simulink model "CartPole_sim"  (R2018b)
settings: Solver=VariableStepAuto  StartTime=0.0  StopTime=100  FixedStep=0.005  MaxStep=0.005  RelTol=1e-3
libraries: neural x90
(part 3 of 3)

== system CartPole_sim/Controller/Layer 3/Delays 1 ==
  "p{3}" : Inport  PortDimensions=48
      mask Display: e = 0.06;c1 = [120 230 180]/255;c2 = ([120 230 180]+0)/(256+128);c3 = ([120 230 180]+128)/(256+128);patch([0 1 1 0],[0 0 1 1],c1);patch([0 1 1 1-e 1-e 0+e],[0 0 1 1-e 0+e 0+e],c2);patch([0 0 1 1-e 0+e 0+e],[0 1 1 1-e 1-e 0+e],c3);plot([0 1 1 0 0],[0 0 1 1 0]);
  mux : Mux  Inputs=1
      mask Display: e = 0.06;c1 = [120 150 230]/255;c2 = ([120 150 230]+0)/383;c3 = ([120 150 230]+128)/383;patch([0 1 1 0],[0 0 1 1],c1);patch([0 1 1 1-e 1-e 0+e],[0 0 1 1-e 0+e 0+e],c2);patch([0 0 1 1-e 0+e 0+e],[0 1 1 1-e 1-e 0+e],c3);plot([0 1 1 0 0],[0 0 1 1 0]);disp('Mux')
  "pd{3,2}" : Outport
      mask Display: e = 0.06;c1 = [120 230 180]/255;c2 = ([120 230 180]+0)/(256+128);c3 = ([120 230 180]+128)/(256+128);patch([0 1 1 0],[0 0 1 1],c1);patch([0 1 1 1-e 1-e 0+e],[0 0 1 1-e 0+e 0+e],c2);patch([0 0 1 1-e 0+e 0+e],[0 1 1 1-e 1-e 0+e],c3);plot([0 1 1 0 0],[0 0 1 1 0]);
  wires:
  mux/1 -> "pd{3,2}"/1
  "p{3}"/1 -> mux/1

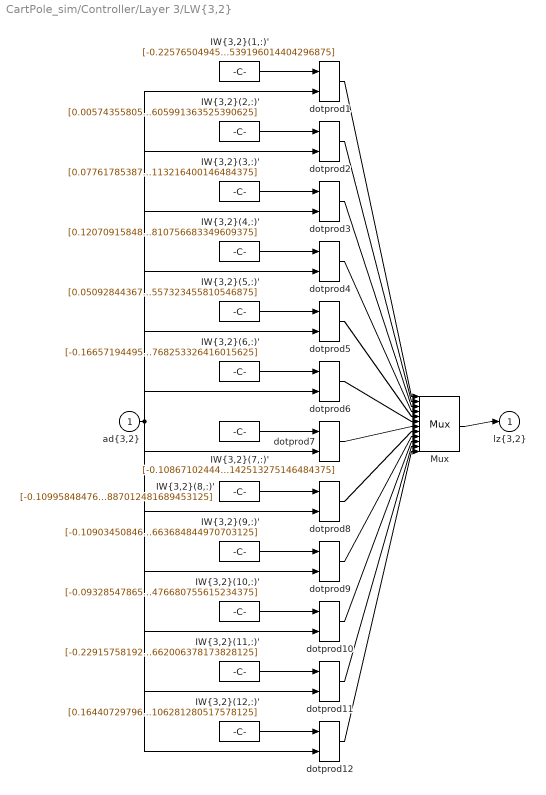
== system CartPole_sim/Controller/Layer 3/LW{3,2} ==
  "ad{3,2}" : Inport  PortDimensions=48
      mask Display: e = 0.06;c1 = [120 230 180]/255;c2 = ([120 230 180]+0)/(256+128);c3 = ([120 230 180]+128)/(256+128);patch([0 1 1 0],[0 0 1 1],c1);patch([0 1 1 1-e 1-e 0+e],[0 0 1 1-e 0+e 0+e],c2);patch([0 0 1 1-e 0+e 0+e],[0 1 1 1-e 1-e 0+e],c3);plot([0 1 1 0 0],[0 0 1 1 0]);
  "IW{3,2}(1,:)'" : Constant  Value=[-0.225765049457550048828125;0.70130741596221923828125;0.73611104488372802734375;0.85522115230560302734375;0.3625166416168212890625;-0.293086946010589599609375;-0.168597280979156494140625;0.62720489501953125;0.7177906036376953125;0.4205109775066375732421875;-0.22078745067119598388671875;0.786495685577392578125;0.598729610443115234375;0.857798099517822265625;-0.19783659279346466064453125;0.5886719226837158203125;0.033965639770030975341796875;0.4852178096771240234375;-0.4360056817531585693359375;-0.13498456776142120361328125;-0.2697825729846954345703125;0.6689045429229736328125;0.02779674716293811798095703125;0.2675172388553619384765625;0.789131581783294677734375;0.59786427021026611328125;0.614151060581207275390625;0.66306316852569580078125;0.59276866912841796875;-0.0609457008540630340576171875;0.62623417377471923828125;-0.18955354392528533935546875;0.755768299102783203125;-0.18641991913318634033203125;0.720268726348876953125;-0.0284832417964935302734375;1.03963196277618408203125;-0.119852729141712188720703125;0.10294115543365478515625;0.4573823511600494384765625;0.23938636481761932373046875;-0.16751043498516082763671875;0.67672908306121826171875;-0.668893158435821533203125;0.2460586130619049072265625;0.44056618213653564453125;0.53306019306182861328125;0.805462539196014404296875]
      mask Display: e = 0.06;c1 = [120 150 230]/255;c2 = ([120 150 230]+0)/383;c3 = ([120 150 230]+128)/383;patch([0 1 1 0],[0 0 1 1],c1);patch([0 1 1 1-e 1-e 0+e],[0 0 1 1-e 0+e 0+e],c2);patch([0 0 1 1-e 0+e 0+e],[0 1 1 1-e 1-e 0+e],c3);plot([0 1 1 0 0],[0 0 1 1 0]);disp('weights');
  "IW{3,2}(10,:)'" : Constant  Value=[-0.093285478651523590087890625;0.3607280552387237548828125;0.58088779449462890625;0.9831249713897705078125;0.71564197540283203125;0.21493326127529144287109375;-0.124086134135723114013671875;0.4439070522785186767578125;0.58334505558013916015625;0.3817100822925567626953125;-0.063464589416980743408203125;-0.2573592662811279296875;0.2025319039821624755859375;0.3065927028656005859375;0.32229793071746826171875;0.4737115204334259033203125;0.02929084934294223785400390625;0.1419357955455780029296875;-0.0101378001272678375244140625;0.3530226647853851318359375;0.707432687282562255859375;0.605476796627044677734375;-0.13292454183101654052734375;-0.0582952834665775299072265625;0.124955832958221435546875;0.519218027591705322265625;0.521830976009368896484375;0.083058618009090423583984375;0.1663186848163604736328125;0.2935204207897186279296875;0.5812957286834716796875;0.22234977781772613525390625;0.7579386234283447265625;0.0754846632480621337890625;0.3434390723705291748046875;-0.1704781055450439453125;0.21832014620304107666015625;-0.30861675739288330078125;-0.279193937778472900390625;0.10558624565601348876953125;0.85374772548675537109375;0.748513400554656982421875;0.553266108036041259765625;-0.24436579644680023193359375;0.08447755873203277587890625;0.507693231105804443359375;0.19571836292743682861328125;0.650114476680755615234375]
      mask Display: e = 0.06;c1 = [120 150 230]/255;c2 = ([120 150 230]+0)/383;c3 = ([120 150 230]+128)/383;patch([0 1 1 0],[0 0 1 1],c1);patch([0 1 1 1-e 1-e 0+e],[0 0 1 1-e 0+e 0+e],c2);patch([0 0 1 1-e 0+e 0+e],[0 1 1 1-e 1-e 0+e],c3);plot([0 1 1 0 0],[0 0 1 1 0]);disp('weights');
  "IW{3,2}(11,:)'" : Constant  Value=[-0.22915758192539215087890625;0.105940572917461395263671875;0.18381464481353759765625;-0.094782888889312744140625;0.17192138731479644775390625;-0.281556427478790283203125;-0.27728307247161865234375;-0.03108619153499603271484375;0.057134740054607391357421875;0.091573022305965423583984375;-0.12182189524173736572265625;0.09163224697113037109375;0.0596763901412487030029296875;0.059483818709850311279296875;0.0422483272850513458251953125;0.2144198119640350341796875;0.253001987934112548828125;-0.22603924572467803955078125;0.027550756931304931640625;0.108232803642749786376953125;0.3021956384181976318359375;-0.34801328182220458984375;0.0536159910261631011962890625;0.007443842478096485137939453125;-0.113824971020221710205078125;-0.11512468755245208740234375;-0.32556056976318359375;0.0549277774989604949951171875;-0.3968221843242645263671875;0.23947632312774658203125;-0.2056002318859100341796875;0.1247394979000091552734375;-0.35302269458770751953125;-0.32575893402099609375;0.32194745540618896484375;-0.084378026425838470458984375;0.06127654016017913818359375;0.16803930699825286865234375;0.14566139876842498779296875;0.0070302230305969715118408203125;-0.09847448766231536865234375;-0.344694912433624267578125;0.2108682692050933837890625;-0.17634133994579315185546875;0.115174196660518646240234375;-0.17366945743560791015625;-0.23996080458164215087890625;-0.3096511662006378173828125]
      mask Display: e = 0.06;c1 = [120 150 230]/255;c2 = ([120 150 230]+0)/383;c3 = ([120 150 230]+128)/383;patch([0 1 1 0],[0 0 1 1],c1);patch([0 1 1 1-e 1-e 0+e],[0 0 1 1-e 0+e 0+e],c2);patch([0 0 1 1-e 0+e 0+e],[0 1 1 1-e 1-e 0+e],c3);plot([0 1 1 0 0],[0 0 1 1 0]);disp('weights');
  "IW{3,2}(12,:)'" : Constant  Value=[0.16440729796886444091796875;-0.095709316432476043701171875;-0.167194426059722900390625;-0.313728511333465576171875;0.087645195424556732177734375;-0.14497192203998565673828125;-0.0050425282679498195648193359375;-0.22736532986164093017578125;0.24480561912059783935546875;-0.14551477134227752685546875;0.24523986876010894775390625;0.08085310459136962890625;-0.073567993938922882080078125;0.18972873687744140625;0.25337803363800048828125;-0.2392151653766632080078125;-0.056765615940093994140625;0.055480085313320159912109375;-0.0636241137981414794921875;-0.104483507573604583740234375;-0.057640530169010162353515625;0.04791681468486785888671875;-0.3014909923076629638671875;-0.1660726070404052734375;0.1237736046314239501953125;-0.25857579708099365234375;-0.3232463300228118896484375;-0.2543390095233917236328125;0.2360977828502655029296875;0.1196926534175872802734375;-0.2703399360179901123046875;0.0864959657192230224609375;0.2298237383365631103515625;0.138822734355926513671875;0.0693146884441375732421875;-0.0826424062252044677734375;0.1139100492000579833984375;-0.0165658928453922271728515625;-0.2953896820545196533203125;-0.250157654285430908203125;-0.2504859268665313720703125;-0.05299697816371917724609375;-0.186982691287994384765625;-0.162210166454315185546875;-0.3076064586639404296875;-0.126573383808135986328125;-0.12438915669918060302734375;-0.339606106281280517578125]
      mask Display: e = 0.06;c1 = [120 150 230]/255;c2 = ([120 150 230]+0)/383;c3 = ([120 150 230]+128)/383;patch([0 1 1 0],[0 0 1 1],c1);patch([0 1 1 1-e 1-e 0+e],[0 0 1 1-e 0+e 0+e],c2);patch([0 0 1 1-e 0+e 0+e],[0 1 1 1-e 1-e 0+e],c3);plot([0 1 1 0 0],[0 0 1 1 0]);disp('weights');
  "IW{3,2}(2,:)'" : Constant  Value=[0.0057435580529272556304931640625;-0.063613593578338623046875;-0.0614121742546558380126953125;-0.2885248363018035888671875;-0.27625179290771484375;0.0465604364871978759765625;0.210648238658905029296875;-0.08427713811397552490234375;-0.145911693572998046875;0.0484735853970050811767578125;-0.037767700850963592529296875;0.13862870633602142333984375;-0.4455624520778656005859375;-0.37608873844146728515625;-0.373650074005126953125;-0.284273922443389892578125;-0.014863868243992328643798828125;-0.12762035429477691650390625;-0.12725473940372467041015625;-0.20327986776828765869140625;-0.2377932965755462646484375;-0.08044274151325225830078125;0.1607999503612518310546875;-0.3193801343441009521484375;0.1244004666805267333984375;-0.2309009730815887451171875;-0.081527270376682281494140625;-0.282345712184906005859375;0.1318136155605316162109375;-0.3154838383197784423828125;-0.2552172243595123291015625;-0.265089333057403564453125;0.123016633093357086181640625;-0.12508480250835418701171875;-0.2878762185573577880859375;0.077459029853343963623046875;-0.2099839150905609130859375;0.0223808549344539642333984375;0.3106609284877777099609375;0.202566623687744140625;0.11093197762966156005859375;0.15283145010471343994140625;0.0318211019039154052734375;-0.2362150251865386962890625;0.1664283275604248046875;-0.3416130542755126953125;0.0929198563098907470703125;0.2078422605991363525390625]
      mask Display: e = 0.06;c1 = [120 150 230]/255;c2 = ([120 150 230]+0)/383;c3 = ([120 150 230]+128)/383;patch([0 1 1 0],[0 0 1 1],c1);patch([0 1 1 1-e 1-e 0+e],[0 0 1 1-e 0+e 0+e],c2);patch([0 0 1 1-e 0+e 0+e],[0 1 1 1-e 1-e 0+e],c3);plot([0 1 1 0 0],[0 0 1 1 0]);disp('weights');
  "IW{3,2}(3,:)'" : Constant  Value=[0.0776178538799285888671875;0.23608161509037017822265625;0.400656223297119140625;0.3066715300083160400390625;0.5607860088348388671875;-0.10452739894390106201171875;-0.1996848583221435546875;-0.07391874492168426513671875;0.2440983951091766357421875;0.2859127223491668701171875;0.181851446628570556640625;-0.566390812397003173828125;0.254243373870849609375;-0.038393653929233551025390625;-0.14987702667713165283203125;0.52229988574981689453125;0.38653004169464111328125;0.0349838696420192718505859375;0.65151679515838623046875;-0.1630626022815704345703125;0.317122280597686767578125;0.87729203701019287109375;0.1295812427997589111328125;-0.2194156348705291748046875;0.3087631165981292724609375;0.3373095691204071044921875;-0.0059780962765216827392578125;0.38896310329437255859375;0.642784178256988525390625;0.123877070844173431396484375;0.50440204143524169921875;0.03245998919010162353515625;0.095179609954357147216796875;-0.067027054727077484130859375;0.588344275951385498046875;0.13531744480133056640625;0.63343536853790283203125;-0.0041498462669551372528076171875;-0.21499086916446685791015625;0.51388394832611083984375;0.70657217502593994140625;0.21739204227924346923828125;0.869004905223846435546875;0.329273223876953125;-0.2585419714450836181640625;0.725928127765655517578125;0.4725751578807830810546875;0.4317859113216400146484375]
      mask Display: e = 0.06;c1 = [120 150 230]/255;c2 = ([120 150 230]+0)/383;c3 = ([120 150 230]+128)/383;patch([0 1 1 0],[0 0 1 1],c1);patch([0 1 1 1-e 1-e 0+e],[0 0 1 1-e 0+e 0+e],c2);patch([0 0 1 1-e 0+e 0+e],[0 1 1 1-e 1-e 0+e],c3);plot([0 1 1 0 0],[0 0 1 1 0]);disp('weights');
  "IW{3,2}(4,:)'" : Constant  Value=[0.120709158480167388916015625;0.01946739666163921356201171875;-0.20635326206684112548828125;-0.2006778419017791748046875;-0.1608820855617523193359375;0.2493370473384857177734375;0.095264874398708343505859375;0.0590558014810085296630859375;0.0524917431175708770751953125;-0.2878700196743011474609375;-0.22221325337886810302734375;0.1907002627849578857421875;-0.3934889137744903564453125;0.08676731586456298828125;0.111214138567447662353515625;0.015520487911999225616455078125;0.0419653095304965972900390625;-0.2015108168125152587890625;0.465694010257720947265625;-0.1469192206859588623046875;-0.16041471064090728759765625;-0.24534873664379119873046875;0.114878714084625244140625;-0.30835545063018798828125;-0.296265184879302978515625;0.1905055940151214599609375;-0.070235051214694976806640625;-0.3958633244037628173828125;-0.078465931117534637451171875;-0.22016370296478271484375;-0.075588651001453399658203125;-0.312045633792877197265625;0.065949432551860809326171875;0.008683224208652973175048828125;0.34296166896820068359375;0.1041338443756103515625;-0.02595026977360248565673828125;-0.20179484784603118896484375;-0.1611983478069305419921875;0.079681120812892913818359375;-0.22468416392803192138671875;0.2698139846324920654296875;0.338930070400238037109375;0.14660227298736572265625;-0.24567271769046783447265625;0.093860089778900146484375;-0.22475038468837738037109375;0.104006610810756683349609375]
      mask Display: e = 0.06;c1 = [120 150 230]/255;c2 = ([120 150 230]+0)/383;c3 = ([120 150 230]+128)/383;patch([0 1 1 0],[0 0 1 1],c1);patch([0 1 1 1-e 1-e 0+e],[0 0 1 1-e 0+e 0+e],c2);patch([0 0 1 1-e 0+e 0+e],[0 1 1 1-e 1-e 0+e],c3);plot([0 1 1 0 0],[0 0 1 1 0]);disp('weights');
  "IW{3,2}(5,:)'" : Constant  Value=[0.0509284436702728271484375;-0.10813932120800018310546875;0.846237242221832275390625;0.548502743244171142578125;0.17196671664714813232421875;0.115305669605731964111328125;0.17061321437358856201171875;-0.010511794127523899078369140625;0.54888880252838134765625;0.296976983547210693359375;0.2747037410736083984375;-0.406587898731231689453125;-0.110211431980133056640625;0.23038510978221893310546875;-0.02488018758594989776611328125;0.4316042363643646240234375;-0.063608609139919281005859375;0.18594552576541900634765625;0.096132762730121612548828125;-0.11069880425930023193359375;0.76139628887176513671875;0.811535537242889404296875;0.0217044539749622344970703125;0.0718050897121429443359375;0.0510326810181140899658203125;0.2666250765323638916015625;0.072972662746906280517578125;0.1536116898059844970703125;0.36417853832244873046875;-0.24053500592708587646484375;0.19662736356258392333984375;-0.15355180203914642333984375;0.6601107120513916015625;-0.2712565958499908447265625;0.67262041568756103515625;0.0377550236880779266357421875;0.3582044541835784912109375;-0.098102755844593048095703125;0.24403761327266693115234375;0.4628359973430633544921875;0.4662868678569793701171875;0.81448459625244140625;0.43295562267303466796875;0.4602414667606353759765625;0.090152136981487274169921875;0.6324546337127685546875;0.288115203380584716796875;0.3198804557323455810546875]
      mask Display: e = 0.06;c1 = [120 150 230]/255;c2 = ([120 150 230]+0)/383;c3 = ([120 150 230]+128)/383;patch([0 1 1 0],[0 0 1 1],c1);patch([0 1 1 1-e 1-e 0+e],[0 0 1 1-e 0+e 0+e],c2);patch([0 0 1 1-e 0+e 0+e],[0 1 1 1-e 1-e 0+e],c3);plot([0 1 1 0 0],[0 0 1 1 0]);disp('weights');
  "IW{3,2}(6,:)'" : Constant  Value=[-0.1665719449520111083984375;0.182851970195770263671875;-0.1930682659149169921875;0.24887974560260772705078125;-0.283345401287078857421875;-0.2073399126529693603515625;0.06374375522136688232421875;-0.23295311629772186279296875;-0.426688611507415771484375;0.083044044673442840576171875;-0.31555879116058349609375;0.4025302827358245849609375;-0.02602317743003368377685546875;0.20263724029064178466796875;-0.194852173328399658203125;-0.296578109264373779296875;0.092311434447765350341796875;0.237321376800537109375;-0.14490391314029693603515625;-0.087759934365749359130859375;0.074599921703338623046875;-0.08056437969207763671875;-0.2687614262104034423828125;0.085790432989597320556640625;0.31562054157257080078125;-0.0375498719513416290283203125;-0.05026900768280029296875;0.23536710441112518310546875;-0.3232409060001373291015625;0.042684264481067657470703125;0.0402791984379291534423828125;0.034206993877887725830078125;-0.17854599654674530029296875;0.24460084736347198486328125;-0.329555809497833251953125;-0.00140616367571055889129638671875;-0.117685638368129730224609375;-0.0323284901678562164306640625;-0.016782738268375396728515625;-0.18480215966701507568359375;-0.38590872287750244140625;-0.0840173065662384033203125;0.17254363000392913818359375;-0.165297031402587890625;0.243590176105499267578125;-0.064210064709186553955078125;0.04639963805675506591796875;0.086828768253326416015625]
      mask Display: e = 0.06;c1 = [120 150 230]/255;c2 = ([120 150 230]+0)/383;c3 = ([120 150 230]+128)/383;patch([0 1 1 0],[0 0 1 1],c1);patch([0 1 1 1-e 1-e 0+e],[0 0 1 1-e 0+e 0+e],c2);patch([0 0 1 1-e 0+e 0+e],[0 1 1 1-e 1-e 0+e],c3);plot([0 1 1 0 0],[0 0 1 1 0]);disp('weights');
  "IW{3,2}(7,:)'" : Constant  Value=[-0.10867102444171905517578125;0.4128165543079376220703125;0.63059222698211669921875;1.07298648357391357421875;0.292224586009979248046875;0.2570346891880035400390625;-0.2520825862884521484375;0.204001247882843017578125;0.71790850162506103515625;0.579679667949676513671875;0.0178261734545230865478515625;-0.4448179900646209716796875;0.483870029449462890625;0.3526272475719451904296875;-0.17523370683193206787109375;0.728261411190032958984375;-0.205432713031768798828125;-0.009472581557929515838623046875;0.009738069958984851837158203125;-0.2126163542270660400390625;0.19845388829708099365234375;0.51429665088653564453125;-0.06766368448734283447265625;0.31298983097076416015625;0.623131215572357177734375;0.610826909542083740234375;0.59944474697113037109375;0.4226538240909576416015625;0.612737596035003662109375;-0.15423603355884552001953125;0.4424777925014495849609375;-0.090688146650791168212890625;0.569411456584930419921875;-0.146714985370635986328125;0.589668929576873779296875;-0.215395748615264892578125;0.92744386196136474609375;-0.024819411337375640869140625;-0.2330188453197479248046875;0.2663786709308624267578125;0.274322092533111572265625;0.0615710504353046417236328125;0.5164601802825927734375;-0.698554933071136474609375;0.3031902611255645751953125;0.09225617349147796630859375;0.5838611125946044921875;0.639142513275146484375]
      mask Display: e = 0.06;c1 = [120 150 230]/255;c2 = ([120 150 230]+0)/383;c3 = ([120 150 230]+128)/383;patch([0 1 1 0],[0 0 1 1],c1);patch([0 1 1 1-e 1-e 0+e],[0 0 1 1-e 0+e 0+e],c2);patch([0 0 1 1-e 0+e 0+e],[0 1 1 1-e 1-e 0+e],c3);plot([0 1 1 0 0],[0 0 1 1 0]);disp('weights');
  "IW{3,2}(8,:)'" : Constant  Value=[-0.10995848476886749267578125;0.7433259487152099609375;0.527641594409942626953125;0.609710276126861572265625;0.562270939350128173828125;-0.3406229317188262939453125;0.3301258981227874755859375;0.646334826946258544921875;0.6849994659423828125;0.276348114013671875;0.1093139350414276123046875;0.221129834651947021484375;0.753832042217254638671875;0.4972431957721710205078125;0.121123097836971282958984375;0.358241856098175048828125;0.13543988764286041259765625;0.14141382277011871337890625;-0.2833416759967803955078125;0.117667324841022491455078125;0.1442694962024688720703125;0.615487158298492431640625;0.1192167699337005615234375;0.01044245995581150054931640625;0.64915740489959716796875;0.2713801562786102294921875;0.658168375492095947265625;0.7554428577423095703125;0.85320007801055908203125;0.0045012016780674457550048828125;0.644239008426666259765625;-0.0504725091159343719482421875;0.595988750457763671875;-0.22417914867401123046875;0.36755478382110595703125;-0.2967093884944915771484375;0.8945713043212890625;-0.102921150624752044677734375;-0.07104603946208953857421875;-0.034781329333782196044921875;0.4639213979244232177734375;0.1595343053340911865234375;0.570801258087158203125;-0.705658733844757080078125;0.15022848546504974365234375;0.53177130222320556640625;0.0694595873355865478515625;0.536775887012481689453125]
      mask Display: e = 0.06;c1 = [120 150 230]/255;c2 = ([120 150 230]+0)/383;c3 = ([120 150 230]+128)/383;patch([0 1 1 0],[0 0 1 1],c1);patch([0 1 1 1-e 1-e 0+e],[0 0 1 1-e 0+e 0+e],c2);patch([0 0 1 1-e 0+e 0+e],[0 1 1 1-e 1-e 0+e],c3);plot([0 1 1 0 0],[0 0 1 1 0]);disp('weights');
  "IW{3,2}(9,:)'" : Constant  Value=[-0.1090345084667205810546875;0.158401787281036376953125;-0.14385612308979034423828125;-0.1813411414623260498046875;0.00181381893344223499298095703125;-0.15125501155853271484375;0.01470577716827392578125;-0.2063058316707611083984375;-0.16525804996490478515625;-0.0644442737102508544921875;-0.265504419803619384765625;0.17381285130977630615234375;-0.4116666615009307861328125;-0.17990852892398834228515625;-0.31012403964996337890625;-0.0989350974559783935546875;-0.23166407644748687744140625;-0.3110125064849853515625;-0.3059598505496978759765625;-0.0589531958103179931640625;0.05852472782135009765625;-0.2704227864742279052734375;-0.0256429016590118408203125;-0.0175074636936187744140625;-0.3467051684856414794921875;-0.0160256326198577880859375;-0.404352664947509765625;0.02101545967161655426025390625;0.2331699430942535400390625;0.2253843843936920166015625;0.0099586546421051025390625;0.1334817111492156982421875;0.16582810878753662109375;0.1585890948772430419921875;0.13788856565952301025390625;-0.3126110136508941650390625;-0.042391359806060791015625;-0.255214869976043701171875;-0.307202875614166259765625;-0.2690750062465667724609375;-0.1166075170040130615234375;-0.2768442630767822265625;-0.01418058574199676513671875;0.070241920650005340576171875;-0.10158611834049224853515625;0.116759471595287322998046875;-0.30962288379669189453125;0.118671126663684844970703125]
      mask Display: e = 0.06;c1 = [120 150 230]/255;c2 = ([120 150 230]+0)/383;c3 = ([120 150 230]+128)/383;patch([0 1 1 0],[0 0 1 1],c1);patch([0 1 1 1-e 1-e 0+e],[0 0 1 1-e 0+e 0+e],c2);patch([0 0 1 1-e 0+e 0+e],[0 1 1 1-e 1-e 0+e],c3);plot([0 1 1 0 0],[0 0 1 1 0]);disp('weights');
  Mux : Mux  Inputs=12
      mask Display: e = 0.06;c1 = [120 150 230]/255;c2 = ([120 150 230]+0)/383;c3 = ([120 150 230]+128)/383;patch([0 1 1 0],[0 0 1 1],c1);patch([0 1 1 1-e 1-e 0+e],[0 0 1 1-e 0+e 0+e],c2);patch([0 0 1 1-e 0+e 0+e],[0 1 1 1-e 1-e 0+e],c3);plot([0 1 1 0 0],[0 0 1 1 0]);disp('Mux');
  dotprod{1..12} (12 alike) : neural/Weight Functions/dotprod
  "lz{3,2}" : Outport
      mask Display: e = 0.06;c1 = [120 230 180]/255;c2 = ([120 230 180]+0)/(256+128);c3 = ([120 230 180]+128)/(256+128);patch([0 1 1 0],[0 0 1 1],c1);patch([0 1 1 1-e 1-e 0+e],[0 0 1 1-e 0+e 0+e],c2);patch([0 0 1 1-e 0+e 0+e],[0 1 1 1-e 1-e 0+e],c3);plot([0 1 1 0 0],[0 0 1 1 0]);
  wires:
  Mux/1 -> "lz{3,2}"/1
  dotprod12/1 -> Mux/12
  "IW{3,2}(12,:)'"/1 -> dotprod12/1
  dotprod11/1 -> Mux/11
  "IW{3,2}(11,:)'"/1 -> dotprod11/1
  dotprod10/1 -> Mux/10
  "IW{3,2}(10,:)'"/1 -> dotprod10/1
  dotprod9/1 -> Mux/9
  "IW{3,2}(9,:)'"/1 -> dotprod9/1
  dotprod8/1 -> Mux/8
  "IW{3,2}(8,:)'"/1 -> dotprod8/1
  dotprod7/1 -> Mux/7
  "IW{3,2}(7,:)'"/1 -> dotprod7/1
  dotprod6/1 -> Mux/6
  "IW{3,2}(6,:)'"/1 -> dotprod6/1
  dotprod5/1 -> Mux/5
  "IW{3,2}(5,:)'"/1 -> dotprod5/1
  dotprod4/1 -> Mux/4
  "IW{3,2}(4,:)'"/1 -> dotprod4/1
  dotprod3/1 -> Mux/3
  "IW{3,2}(3,:)'"/1 -> dotprod3/1
  dotprod2/1 -> Mux/2
  "IW{3,2}(2,:)'"/1 -> dotprod2/1
  dotprod1/1 -> Mux/1
  "ad{3,2}"/1 -> dotprod12/2, dotprod11/2, dotprod10/2, dotprod9/2, dotprod8/2, dotprod7/2, dotprod6/2, dotprod5/2, dotprod4/2, dotprod3/2, dotprod2/2, dotprod1/2
  "IW{3,2}(1,:)'"/1 -> dotprod1/1

== system CartPole_sim/Controller/Layer 4/Delays 1 ==
  "p{4}" : Inport  PortDimensions=12
      mask Display: e = 0.06;c1 = [120 230 180]/255;c2 = ([120 230 180]+0)/(256+128);c3 = ([120 230 180]+128)/(256+128);patch([0 1 1 0],[0 0 1 1],c1);patch([0 1 1 1-e 1-e 0+e],[0 0 1 1-e 0+e 0+e],c2);patch([0 0 1 1-e 0+e 0+e],[0 1 1 1-e 1-e 0+e],c3);plot([0 1 1 0 0],[0 0 1 1 0]);
  mux : Mux  Inputs=1
      mask Display: e = 0.06;c1 = [120 150 230]/255;c2 = ([120 150 230]+0)/383;c3 = ([120 150 230]+128)/383;patch([0 1 1 0],[0 0 1 1],c1);patch([0 1 1 1-e 1-e 0+e],[0 0 1 1-e 0+e 0+e],c2);patch([0 0 1 1-e 0+e 0+e],[0 1 1 1-e 1-e 0+e],c3);plot([0 1 1 0 0],[0 0 1 1 0]);disp('Mux')
  "pd{4,3}" : Outport
      mask Display: e = 0.06;c1 = [120 230 180]/255;c2 = ([120 230 180]+0)/(256+128);c3 = ([120 230 180]+128)/(256+128);patch([0 1 1 0],[0 0 1 1],c1);patch([0 1 1 1-e 1-e 0+e],[0 0 1 1-e 0+e 0+e],c2);patch([0 0 1 1-e 0+e 0+e],[0 1 1 1-e 1-e 0+e],c3);plot([0 1 1 0 0],[0 0 1 1 0]);
  wires:
  mux/1 -> "pd{4,3}"/1
  "p{4}"/1 -> mux/1

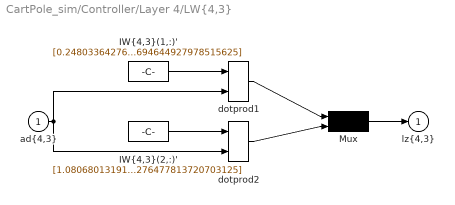
== system CartPole_sim/Controller/Layer 4/LW{4,3} ==
  "ad{4,3}" : Inport  PortDimensions=12
      mask Display: e = 0.06;c1 = [120 230 180]/255;c2 = ([120 230 180]+0)/(256+128);c3 = ([120 230 180]+128)/(256+128);patch([0 1 1 0],[0 0 1 1],c1);patch([0 1 1 1-e 1-e 0+e],[0 0 1 1-e 0+e 0+e],c2);patch([0 0 1 1-e 0+e 0+e],[0 1 1 1-e 1-e 0+e],c3);plot([0 1 1 0 0],[0 0 1 1 0]);
  "IW{4,3}(1,:)'" : Constant  Value=[0.24803364276885986328125;-0.470801174640655517578125;0.98562896251678466796875;-0.0494449436664581298828125;0.809553563594818115234375;-0.38018310070037841796875;0.828412711620330810546875;0.287147343158721923828125;-0.506376564502716064453125;0.60969340801239013671875;0.19456170499324798583984375;-0.2804962694644927978515625]
      mask Display: e = 0.06;c1 = [120 150 230]/255;c2 = ([120 150 230]+0)/383;c3 = ([120 150 230]+128)/383;patch([0 1 1 0],[0 0 1 1],c1);patch([0 1 1 1-e 1-e 0+e],[0 0 1 1-e 0+e 0+e],c2);patch([0 0 1 1-e 0+e 0+e],[0 1 1 1-e 1-e 0+e],c3);plot([0 1 1 0 0],[0 0 1 1 0]);disp('weights');
  "IW{4,3}(2,:)'" : Constant  Value=[1.0806801319122314453125;0.433215558528900146484375;0.21181547641754150390625;-0.69721281528472900390625;0.171673953533172607421875;-0.472988784313201904296875;0.962528645992279052734375;0.607547104358673095703125;0.29869091510772705078125;0.3790217936038970947265625;-0.585186481475830078125;0.22761817276477813720703125]
      mask Display: e = 0.06;c1 = [120 150 230]/255;c2 = ([120 150 230]+0)/383;c3 = ([120 150 230]+128)/383;patch([0 1 1 0],[0 0 1 1],c1);patch([0 1 1 1-e 1-e 0+e],[0 0 1 1-e 0+e 0+e],c2);patch([0 0 1 1-e 0+e 0+e],[0 1 1 1-e 1-e 0+e],c3);plot([0 1 1 0 0],[0 0 1 1 0]);disp('weights');
  Mux : Mux  Inputs=2
      mask Display: e = 0.06;c1 = [120 150 230]/255;c2 = ([120 150 230]+0)/383;c3 = ([120 150 230]+128)/383;patch([0 1 1 0],[0 0 1 1],c1);patch([0 1 1 1-e 1-e 0+e],[0 0 1 1-e 0+e 0+e],c2);patch([0 0 1 1-e 0+e 0+e],[0 1 1 1-e 1-e 0+e],c3);plot([0 1 1 0 0],[0 0 1 1 0]);disp('Mux');
  dotprod1 : neural/Weight Functions/dotprod
  dotprod2 : neural/Weight Functions/dotprod
  "lz{4,3}" : Outport
      mask Display: e = 0.06;c1 = [120 230 180]/255;c2 = ([120 230 180]+0)/(256+128);c3 = ([120 230 180]+128)/(256+128);patch([0 1 1 0],[0 0 1 1],c1);patch([0 1 1 1-e 1-e 0+e],[0 0 1 1-e 0+e 0+e],c2);patch([0 0 1 1-e 0+e 0+e],[0 1 1 1-e 1-e 0+e],c3);plot([0 1 1 0 0],[0 0 1 1 0]);
  wires:
  Mux/1 -> "lz{4,3}"/1
  dotprod2/1 -> Mux/2
  "IW{4,3}(2,:)'"/1 -> dotprod2/1
  dotprod1/1 -> Mux/1
  "ad{4,3}"/1 -> dotprod2/2, dotprod1/2
  "IW{4,3}(1,:)'"/1 -> dotprod1/1

== matlab function CartPole_sim/MATLAB Function ==
  data: u input; y output
function y = fcn(u)
    if u(1)>u(2)
        x = -10;
    else
        x = 10;
    end
y = x;

== stateflow chart CartPole_sim/Cart-Pole plant ==
  settings: updateMethod=CONTINUOUS
  state Moving
    du:
    x_dot = v;
    theta_dot = omega;
    v_dot =((u + 0.05*omega*omega*sin(theta))/1.1)-0.05*(9.8*sin(theta)-cos(theta)*((u+0.05*omega*omega*sin(theta))/1.1))/(0.5*(4/3-0.1*cos(theta)*cos(theta)/1.1))*cos(theta)/1.1;
    omega_dot = (9.8*sin(theta)-cos(theta)*((u+0.05*omega*omega*sin(theta))/1.1))/(0.5*(4/3-0.1*cos(theta)*cos(theta)/1.1));
    x_out = x;
    theta_out=theta;
    v_out = v;
    omega_out = omega;
  (default) -> Moving : {x=0;
      | theta = 0.01;
      | omega = 0;
      | v = 0;}
  data: x local; theta local; omega local; v local; x_out output; theta_out output; v_out output; omega_out output; u input
  data x settings: updateMethod=SF_CONTINUOUS_TIME_DATA
  data theta settings: updateMethod=SF_CONTINUOUS_TIME_DATA
  data omega settings: updateMethod=SF_CONTINUOUS_TIME_DATA
  data v settings: updateMethod=SF_CONTINUOUS_TIME_DATA
